simulink model "N扇区"  (R2024b)
settings: Solver=VariableStepAuto  StartTime=0.0  StopTime=10.0  RelTol=1e-3
settings Model: Creator=86195  LastModifiedBy=86195

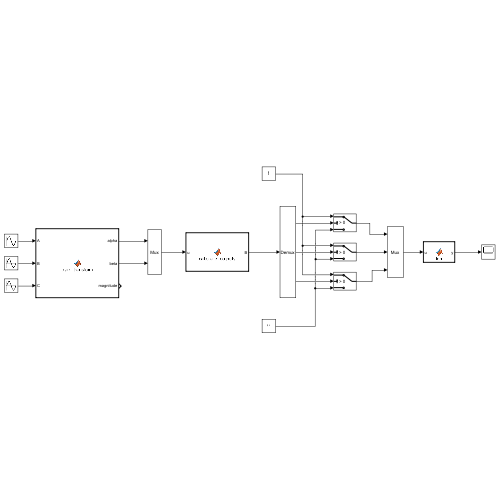
[thumbnail: Simulink's stored preview of the top-level diagram]
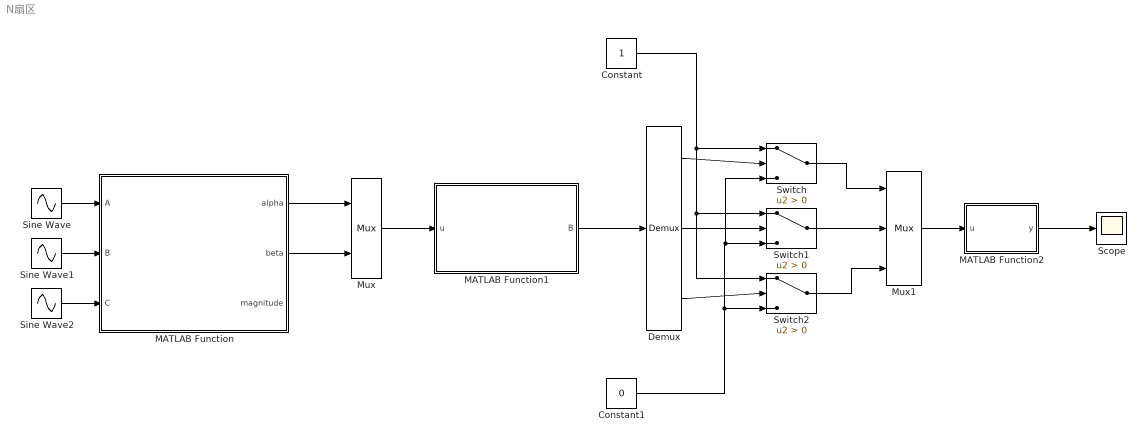
== system N扇区 ==
  Constant : Constant
  Constant1 : Constant  Value=0
  Demux : Demux  Outputs=3
      settings: DisplayOption=none
  MATLAB Function : MATLAB Function  TreatAsAtomicUnit=on
  MATLAB Function1 : MATLAB Function  TreatAsAtomicUnit=on
  MATLAB Function2 : MATLAB Function  TreatAsAtomicUnit=on
  Mux : Mux  Inputs=2
  Mux1 : Mux  Inputs=3
  Scope : Scope
  Sine Wave : Sin  Amplitude=220  Frequency=50*2*pi  SampleTime=0
  Sine Wave1 : Sin  Amplitude=220  Frequency=50*2*pi  Phase=120/180*pi  SampleTime=0
  Sine Wave2 : Sin  Amplitude=220  Frequency=50*2*pi  Phase=-120/180*pi  SampleTime=0
  Switch : Switch  Criteria=u2 > Threshold  SaturateOnIntegerOverflow=off  InputSameDT=off
  Switch1 : Switch  Criteria=u2 > Threshold  SaturateOnIntegerOverflow=off  InputSameDT=off
  Switch2 : Switch  Criteria=u2 > Threshold  SaturateOnIntegerOverflow=off  InputSameDT=off
  wires:
  Sine Wave2/1 -> MATLAB Function/3(C)
  Sine Wave/1 -> MATLAB Function/1(A)
  Sine Wave1/1 -> MATLAB Function/2(B)
  MATLAB Function/1(alpha) -> Mux/1
  MATLAB Function/2(beta) -> Mux/2
  Mux/1 -> MATLAB Function1/1(u)
  MATLAB Function1/1(B) -> Demux/1
  Demux/1 -> Switch/2
  Demux/2 -> Switch1/2
  Demux/3 -> Switch2/2
  Switch/1 -> Mux1/1
  Switch1/1 -> Mux1/2
  Switch2/1 -> Mux1/3
  Constant/1 -> Switch/1, Switch1/1, Switch2/1
  Constant1/1 -> Switch/3, Switch1/3, Switch2/3
  Mux1/1 -> MATLAB Function2/1(u)
  MATLAB Function2/1(y) -> Scope/1

== matlab function N扇区/MATLAB Function1 ==
  data: u input; B output
function B = calculate_outputs(u)
    % 假设 u 是一个至少包含2个元素的向量
    % u(1) 对应图中的 u[1]
    % u(2) 对应图中的 u[2]
    
    % 为了代码更清晰，可以先提取 u(1) 和 u(2)
    u1 = u(1);
    u2 = u(2);
    
    % B0 的计算
    B0 = u2;
    
    % B1 的计算
    k = sqrt(3/4); % 预先计算常量，也可以写作 sqrt(3)/2
    B1 = u1 * k - 0.5 * u2;
    
    % B2 的计算
    B2 = -u1 * k - 0.5 * u2;
    
    % 将结果B0, B1, B2合并为一个列向量
    B = [B0; B1; B2];
end

== matlab function N扇区/MATLAB Function ==
  data: A input; alpha output; B input; C input; beta output; magnitude output
function [alpha, beta, magnitude] = clark_transform(A, B, C)
% 恒定幅值Clark变换矩阵
T = (2/3) * [1,  -1/2,      -1/2;
            0,  sqrt(3)/2, -sqrt(3)/2];
% 将三相信号转换为列向量
abc = [A; B; C];
% 应用Clark变换
alpha_beta = T * abc;
% 提取alpha和beta分量
alpha = alpha_beta(1);
beta = alpha_beta(2);
% 计算合成矢量的幅值
magnitude = sqrt(alpha^2 + beta^2);
end

== matlab function N扇区/MATLAB Function2 ==
  data: u input; y output
function y = fcn(u)

y = 4*u(3)+2*u(2)+u(1);
